simulink model "stwart_platform_model"  (R2026a)
settings: Solver=VariableStepAuto
undefined symbols (not defined in the file): X, Y, Z
libraries: sm_lib x64, nesl_utility x7
(part 1 of 3)
settings Model: Creator=Ojas Padhye  LastModifiedBy=Ojas Padhye

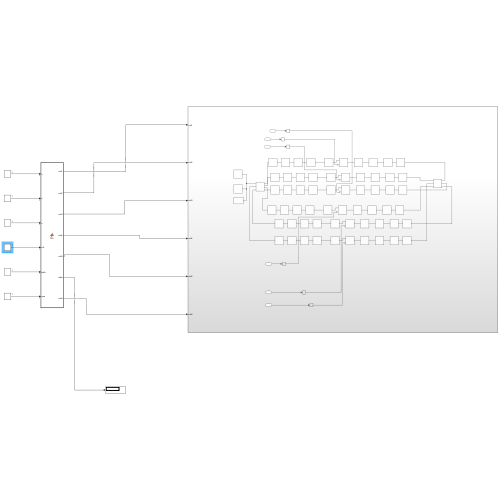
[thumbnail: Simulink's stored preview of the top-level diagram]
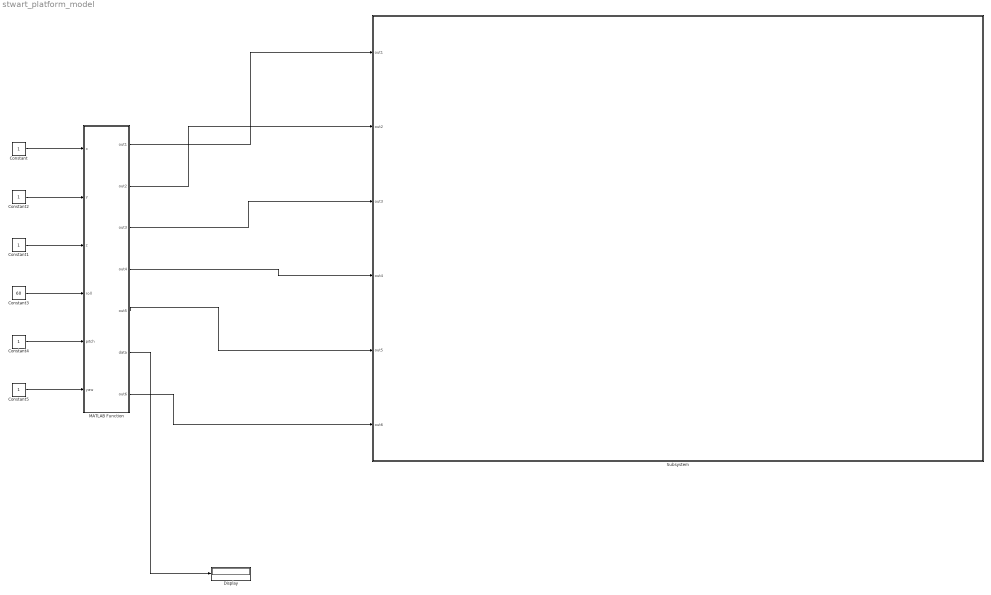
== system stwart_platform_model ==
  Constant{,1..2,4..5} (5 alike) : Constant
  Constant3 : Constant  Value=60
  Display : Display
  MATLAB Function : MATLAB Function  TreatAsAtomicUnit=on
  Subsystem : Subsystem
  wires:
  MATLAB Function/5(out5) -> Subsystem/5(out5)
  MATLAB Function/4(out4) -> Subsystem/4(out4)
  MATLAB Function/3(out3) -> Subsystem/3(out3)
  MATLAB Function/7(out6) -> Subsystem/6(out6)
  MATLAB Function/1(out1) -> Subsystem/1(out1)
  MATLAB Function/2(out2) -> Subsystem/2(out2)
  MATLAB Function/6(data) -> Display/1
  Constant/1 -> MATLAB Function/1(x)
  Constant2/1 -> MATLAB Function/2(y)
  Constant1/1 -> MATLAB Function/3(z)
  Constant3/1 -> MATLAB Function/4(roll)
  Constant4/1 -> MATLAB Function/5(pitch)
  Constant5/1 -> MATLAB Function/6(yaw)
